simulink model "ACMCprogress22bfianl"  (R2022b)
settings: Solver=ode4  StartTime=0.0  StopTime=0.5  FixedStep=1e-7  RelTol=1e-3
libraries: spsSeriesRLCBranchLib x3, spsVoltageMeasurementLib x2, spsControlledVoltageSourceLib x1, spsCurrentMeasurementLib x1, spsDiodeLib x1, spsMosfetLib x1, simulink x1, spspowerguiLib x1
settings Model: Creator=Kashib Khan  LastModifiedBy=saura
settings OptimizationCC: ReuseModelBlockBuffer=on
settings RTWCC: GPUComputeCapability=5.0

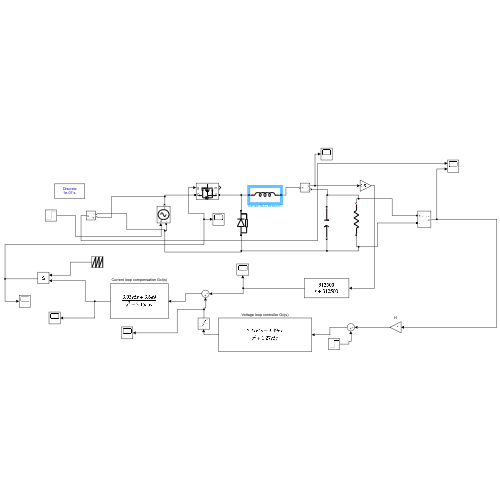
[thumbnail: Simulink's stored preview of the top-level diagram]
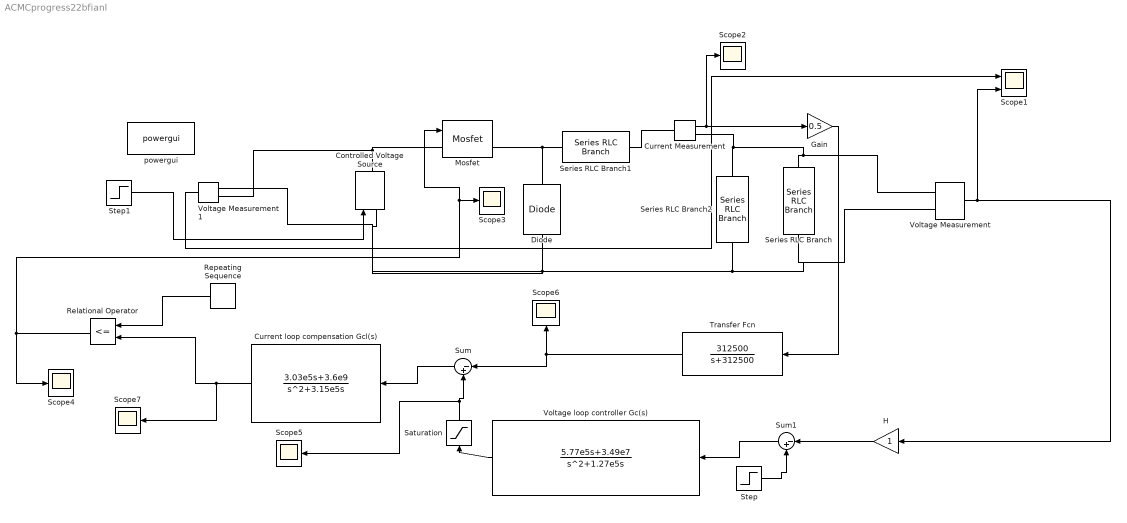
== system ACMCprogress22bfianl ==
  Controlled Voltage Source : spsControlledVoltageSourceLib/Controlled Voltage Source  Initialize=on  Source_Type=DC  Amplitude=10  Phase=0  Frequency=0  Measurements=None
  Current Measurement : spsCurrentMeasurementLib/Current Measurement  PhasorSimulation=off  OutputType=Complex  PSBequivalent=0
  Current loop compensation Gcl(s) : TransferFcn  Numerator=[3.03e5 3.6e9]  Denominator=[1 3.15e5 0]
  Diode : spsDiodeLib/Diode  Ron=0.22  Lon=0  Vf=0.8  IC=0  UseSnubber=0  Rs=500  Cs=250e-9  Measurements=off
  Gain : Gain  Gain=0.5
  H : Gain
  Mosfet : spsMosfetLib/Mosfet  Ron=0.11  Lon=0  Rd=0.01  Vfd=0  IC=0  Rs=1e5  Cs=inf  Measurements=on
  Relational Operator : RelationalOperator  Operator=<=  OutDataTypeStr=boolean  RndMeth=Simplest  InputSameDT=off
  Repeating Sequence : simulink/Sources/Repeating Sequence  rep_seq_t=[0 6.67e-6]  rep_seq_y=[0 1.88]
  Saturation : Saturate  UpperLimit=10  LowerLimit=0
  Scope1 : Scope  NumInputPorts=2
  Scope{2..7} (6 alike) : Scope
  Series RLC Branch : spsSeriesRLCBranchLib/Series RLC Branch  LConnTagsString=__new0  RConnTagsString=__new0  BranchType=R  Resistance=5  Inductance=1e-3  SetiL0=off  InitialCurrent=0  Capacitance=1e-6  Setx0=off  InitialVoltage=0  Measurements=None
  Series RLC Branch1 : spsSeriesRLCBranchLib/Series RLC Branch  LConnTagsString=__new0  RConnTagsString=__new0  BranchType=L  Resistance=1.2  Inductance=2e-5  SetiL0=off  InitialCurrent=0  Capacitance=1e-6  Setx0=off  InitialVoltage=0  Measurements=None
  Series RLC Branch2 : spsSeriesRLCBranchLib/Series RLC Branch  LConnTagsString=__new0  RConnTagsString=__new0  BranchType=C  Resistance=1  Inductance=1e-3  SetiL0=off  InitialCurrent=0  Capacitance=330e-6  Setx0=off  InitialVoltage=0  Measurements=None
  Step : Step  Time=0.1  Before=4  After=6  SampleTime=0
  Step1 : Step  Time=0  Before=10  After=10  SampleTime=0
  Sum : Sum  Inputs=|-+
  Sum1 : Sum  Inputs=|-+
  Transfer Fcn : TransferFcn  Numerator=[312500]  Denominator=[1 312500]
  Voltage Measurement : spsVoltageMeasurementLib/Voltage Measurement  PhasorSimulation=off  OutputType=Complex  PSBequivalent=0
  Voltage Measurement1 : spsVoltageMeasurementLib/Voltage Measurement  PhasorSimulation=off  OutputType=Complex  PSBequivalent=0
  Voltage loop controller Gc(s) : TransferFcn  Numerator="[5.77e5  3.49e7]"  Denominator=[1 1.27e5 0]
  powergui : spspowerguiLib/powergui  Priority=1  SimulationMode=Discrete  SampleTime=1e-7  frequency=60  Iterations=50  frequencyindice=0  Pbase=100e6  ErrMax=1e-4  UnitsV=kV  UnitsW=MW  buscounter=0  FunctionMessages=off  echomessages=off  EnableUseOfTLC=off  CurrentSourceSwitches=off  DisableSnubberDevices=off  DisableRonSwitches=off  DisableVfSwitches=off  DisplayEquations=off  AutomaticDiscreteSolvers=off  SolverType=Tustin/Backward Euler (TBE)  Interpol=off  ExternalGateDelay=off  methode=off  Ts=100  x0status=blocks  SPID=on  SwTol=0  HookPort=off  NonlinearTolerance=1e-4  nMaxIteration=100  ContinueOnMaxIteration=off  RestoreLinks=warning  ResistiveCurrentMeasurement=off  Frange=[0:2:500]  Ylog=off  Xlog=on  ShowGrid=off  save=off  variable=ZData  structure=0  ZoomFFT=off  StartTime=0.0  cycles=1  DisplayStyle=1  fundamental=60  FreqAxis=off  MaxFrequency=1000  frequencyindicesteady=1  RmsSteady=1  display=off
  wires:
  Current Measurement/1 -> Gain/1, Scope2/1
  Voltage Measurement/1 -> Scope1/2, H/1
  H/1 -> Sum1/1
  Step/1 -> Sum1/2
  Sum1/1 -> Voltage loop controller Gc(s)/1
  Relational Operator/1 -> Scope3/1, Mosfet/1, Scope4/1
  Sum/1 -> Current loop compensation Gcl(s)/1
  Current loop compensation Gcl(s)/1 -> Scope7/1, Relational Operator/2
  Repeating Sequence/1 -> Relational Operator/1
  Gain/1 -> Transfer Fcn/1
  Saturation/1 -> Sum/2, Scope5/1
  Voltage loop controller Gc(s)/1 -> Saturation/1
  Transfer Fcn/1 -> Sum/1, Scope6/1
  Step1/1 -> Controlled Voltage Source/1
  Voltage Measurement1/1 -> Scope1/1
  connections:
  Controlled Voltage Source/RConn1 -- Voltage Measurement1/LConn1 -- Mosfet/LConn1
  Mosfet/RConn1 -- Series RLC Branch1/LConn1 -- Diode/RConn1
  Voltage Measurement/LConn2 -- Series RLC Branch/RConn1 -- Series RLC Branch2/RConn1 -- Voltage Measurement1/LConn2 -- Controlled Voltage Source/LConn1 -- Diode/LConn1
  Series RLC Branch2/LConn1 -- Current Measurement/RConn1 -- Voltage Measurement/LConn1 -- Series RLC Branch/LConn1
  Series RLC Branch1/RConn1 -- Current Measurement/LConn1
